simulink model "AD1939_Avalon_Stream_Processing_v1"  (R2018b)
settings: Solver=FixedStepDiscrete  StartTime=0.0  StopTime=stop_time  RelTol=1e-3
InitFcn:
  | DataPlane_callback_init
StopFcn:
  | DataPlane_callback_stop
undefined symbols (not defined in the file or in its folder): F_bits, Ts_system, W_bits
libraries: hdlsllib x18, simulink x5, dspsrcs4 x4, dsphdlfiltering x2
(part 1 of 2)
settings Model: Creator=Ross  LastModifiedBy=trevor
settings OptimizationCC: BlockReduction=off  ConditionallyExecuteInputs=off  DefaultParameterBehavior=Inlined
settings DebuggingCC: AlgebraicLoopMsg=error  SingleTaskRateTransMsg=error  LibraryContextMissingDiagnostic=none
settings HardwareCC: ProdBitPerPointer=32  ProdBitPerSizeT=32  ProdBitPerPtrDiffT=32  ProdLargestAtomicFloat=None  ProdIntDivRoundTo=Undefined  ProdEndianess=Unspecified  ProdWordSize=32  ProdHWDeviceType=ASIC/FPGA->ASIC/FPGA  TargetBitPerLong=64  TargetBitPerPointer=64  TargetBitPerSizeT=64  TargetBitPerPtrDiffT=64  TargetLongLongMode=on  TargetIntDivRoundTo=Zero  TargetEndianess=LittleEndian  TargetWordSize=64  TargetHWDeviceType=Custom Processor->MATLAB Host Computer  ProdEqTarget=off
settings SFSimCC: SimUseLocalCustomCode=off
settings RTWCC: RTWUseLocalCustomCode=off

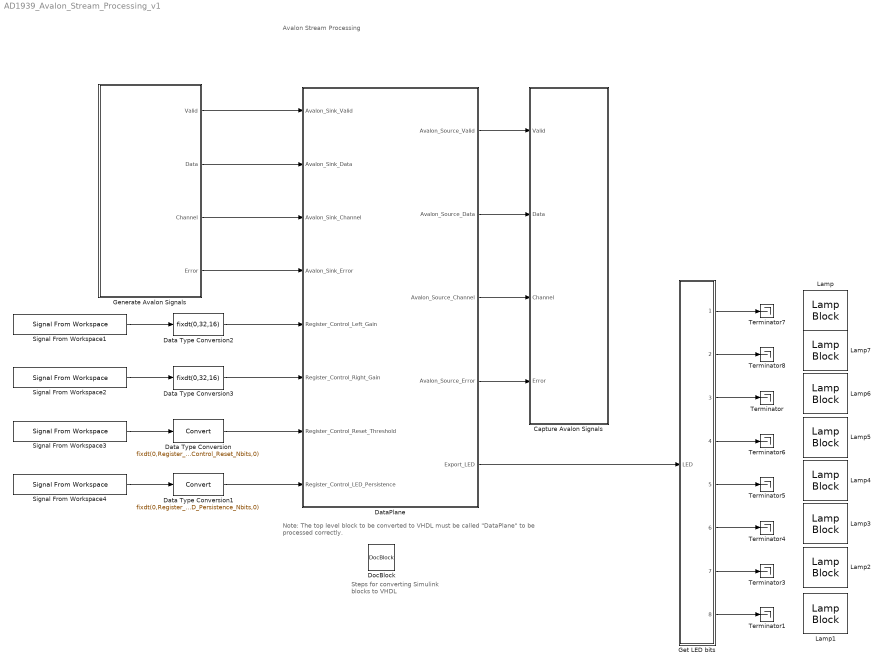
== system AD1939_Avalon_Stream_Processing_v1 ==
  note: Note:  The top level block to be converted to VHDL must be called "DataPlane"
      | to be processed correctly.
  note: Steps for converting
      | Simulink blocks
      | to VHDL
  note: Avalon Stream Processing
  Capture Avalon Signals : Subsystem
  Data Type Conversion : DataTypeConversion  OutDataTypeStr=fixdt(0,Register_Control_Reset_Nbits,0)
  Data Type Conversion1 : DataTypeConversion  OutDataTypeStr=fixdt(0,Register_Control_LED_Persistence_Nbits,0)
  Data Type Conversion2 : DataTypeConversion  OutDataTypeStr=fixdt(0,32,16)
  Data Type Conversion3 : DataTypeConversion  OutDataTypeStr=fixdt(0,32,16)
  DataPlane : Subsystem  TreatAsAtomicUnit=on
  DocBlock : simulink/Model-Wide Utilities/DocBlock  DocumentType=HTML
  Generate Avalon Signals : Subsystem
  Get LED bits : Subsystem
  Lamp : LampBlock  WebBlockId=954
  Lamp1 : LampBlock  WebBlockId=955
  Lamp2 : LampBlock  WebBlockId=956
  Lamp3 : LampBlock  WebBlockId=957
  Lamp4 : LampBlock  WebBlockId=958
  Lamp5 : LampBlock  WebBlockId=959
  Lamp6 : LampBlock  WebBlockId=960
  Lamp7 : LampBlock  WebBlockId=961
  Signal From Workspace1 : dspsrcs4/Signal From Workspace  X=Register_Control_Left_Gain  Ts=Ts_system  nsamps=1  OutputAfterFinalValue=Holding final value  ignoreOrWarnInputAndFrameLengths=off  OutputFrames=off
  Signal From Workspace2 : dspsrcs4/Signal From Workspace  X=Register_Control_Right_Gain  Ts=Ts_system  nsamps=1  OutputAfterFinalValue=Holding final value  ignoreOrWarnInputAndFrameLengths=off  OutputFrames=off
  Signal From Workspace3 : dspsrcs4/Signal From Workspace  X=Register_Control_Reset_Threshold  Ts=Ts_system  nsamps=1  OutputAfterFinalValue=Holding final value  ignoreOrWarnInputAndFrameLengths=off  OutputFrames=off
  Signal From Workspace4 : dspsrcs4/Signal From Workspace  X=Register_Control_LED_Persistence  Ts=Ts_system  nsamps=1  OutputAfterFinalValue=Holding final value  ignoreOrWarnInputAndFrameLengths=off  OutputFrames=off
  Terminator{,1,3..8} (8 alike) : Terminator
  wires:
  Generate Avalon Signals/2(Data) -> DataPlane/2(Avalon_Sink_Data)
  Generate Avalon Signals/1(Valid) -> DataPlane/1(Avalon_Sink_Valid)
  Generate Avalon Signals/3(Channel) -> DataPlane/3(Avalon_Sink_Channel)
  Generate Avalon Signals/4(Error) -> DataPlane/4(Avalon_Sink_Error)
  DataPlane/2(Avalon_Source_Data) -> Capture Avalon Signals/2(Data)
  DataPlane/1(Avalon_Source_Valid) -> Capture Avalon Signals/1(Valid)
  DataPlane/3(Avalon_Source_Channel) -> Capture Avalon Signals/3(Channel)
  DataPlane/4(Avalon_Source_Error) -> Capture Avalon Signals/4(Error)
  Signal From Workspace3/1 -> Data Type Conversion/1
  Signal From Workspace4/1 -> Data Type Conversion1/1
  Data Type Conversion/1 -> DataPlane/7(Register_Control_Reset_Threshold)
  Data Type Conversion1/1 -> DataPlane/8(Register_Control_LED_Persistence)
  Get LED bits/7(LED_1) -> Terminator3/1
  Get LED bits/4(LED_4) -> Terminator6/1
  Get LED bits/1(LED_7) -> Terminator7/1
  Get LED bits/6(LED_2) -> Terminator4/1
  Get LED bits/2(LED_6) -> Terminator8/1
  Get LED bits/8(LED_0) -> Terminator1/1
  Get LED bits/5(LED_3) -> Terminator5/1
  Get LED bits/3(LED_5) -> Terminator/1
  DataPlane/5(Export_LED) -> Get LED bits/1(LED)
  Signal From Workspace1/1 -> Data Type Conversion2/1
  Signal From Workspace2/1 -> Data Type Conversion3/1
  Data Type Conversion2/1 -> DataPlane/5(Register_Control_Left_Gain)
  Data Type Conversion3/1 -> DataPlane/6(Register_Control_Right_Gain)

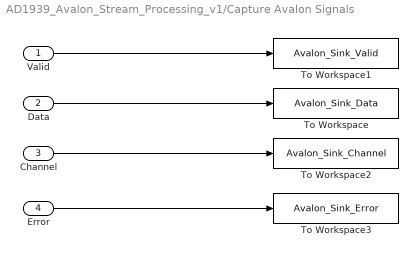
== system AD1939_Avalon_Stream_Processing_v1/Capture Avalon Signals ==
  Valid : Inport
  Data : Inport  Port=2
  Channel : Inport  Port=3
  Error : Inport  Port=4
  To Workspace : ToWorkspace  VariableName=Avalon_Sink_Data  SaveFormat=Timeseries  SampleTime=-1
  To Workspace1 : ToWorkspace  VariableName=Avalon_Sink_Valid  SaveFormat=Timeseries  SampleTime=-1
  To Workspace2 : ToWorkspace  VariableName=Avalon_Sink_Channel  SaveFormat=Timeseries  SampleTime=-1
  To Workspace3 : ToWorkspace  VariableName=Avalon_Sink_Error  SaveFormat=Timeseries  SampleTime=-1
  wires:
  Data/1 -> To Workspace/1
  Valid/1 -> To Workspace1/1
  Error/1 -> To Workspace3/1
  Channel/1 -> To Workspace2/1

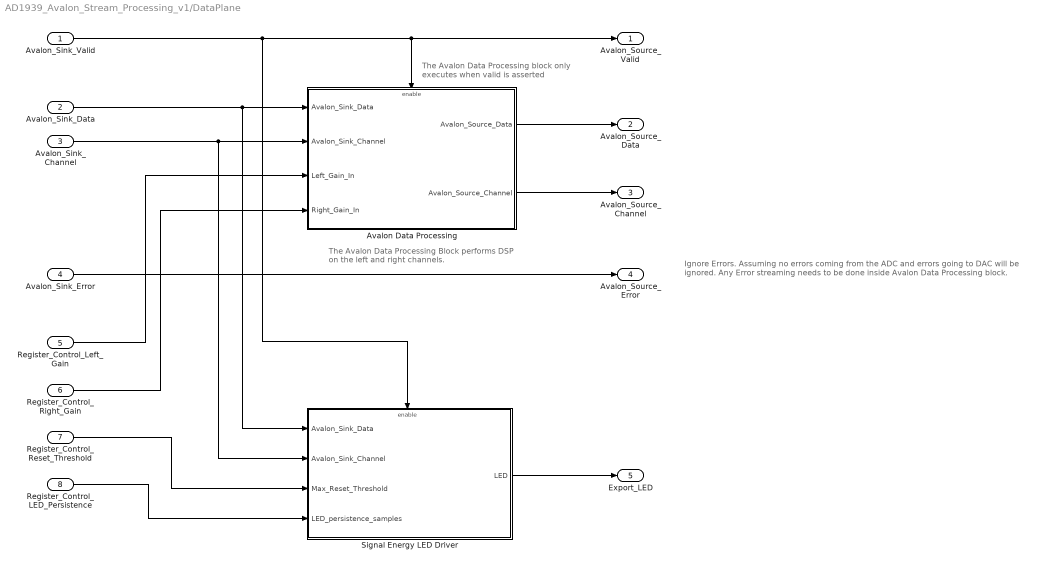
== system AD1939_Avalon_Stream_Processing_v1/DataPlane ==
  note: The Avalon Data Processing Block
      | performs DSP on the left and right channels.
  note: The Avalon Data Processing block
      | only executes when valid is asserted
  note: Ignore Errors.
      | Assuming no errors coming from the ADC and errors going to DAC will be ignored.
      | Any Error streaming needs to be done inside Avalon Data Processing block.
  Avalon_Sink_Valid : Inport
  Avalon_Sink_Data : Inport  Port=2
  Avalon_Sink_Channel : Inport  Port=3
  Avalon_Sink_Error : Inport  Port=4
  Register_Control_Left_Gain : Inport  Port=5
  Register_Control_Right_Gain : Inport  Port=6
  Register_Control_Reset_Threshold : Inport  Port=7
  Register_Control_LED_Persistence : Inport  Port=8
  Avalon Data Processing : Subsystem  TreatAsAtomicUnit=on
  Signal Energy LED Driver : Subsystem  TreatAsAtomicUnit=on
  Avalon_Source_Valid : Outport
  Avalon_Source_Data : Outport  Port=2
  Avalon_Source_Channel : Outport  Port=3
  Avalon_Source_Error : Outport  Port=4
  Export_LED : Outport  Port=5  InitialOutput=0
  wires:
  Avalon_Sink_Channel/1 -> Signal Energy LED Driver/2(Avalon_Sink_Channel), Avalon Data Processing/2(Avalon_Sink_Channel)
  Avalon_Sink_Error/1 -> Avalon_Source_Error/1
  Avalon Data Processing/1(Avalon_Source_Data) -> Avalon_Source_Data/1
  Avalon_Sink_Valid/1 -> Signal Energy LED Driver/Enable, Avalon Data Processing/Enable, Avalon_Source_Valid/1
  Avalon_Sink_Data/1 -> Signal Energy LED Driver/1(Avalon_Sink_Data), Avalon Data Processing/1(Avalon_Sink_Data)
  Avalon Data Processing/2(Avalon_Source_Channel) -> Avalon_Source_Channel/1
  Register_Control_Right_Gain/1 -> Avalon Data Processing/4(Right_Gain_In)
  Register_Control_Left_Gain/1 -> Avalon Data Processing/3(Left_Gain_In)
  Signal Energy LED Driver/1(LED) -> Export_LED/1
  Register_Control_Reset_Threshold/1 -> Signal Energy LED Driver/3(Max_Reset_Threshold)
  Register_Control_LED_Persistence/1 -> Signal Energy LED Driver/4(LED_persistence_samples)

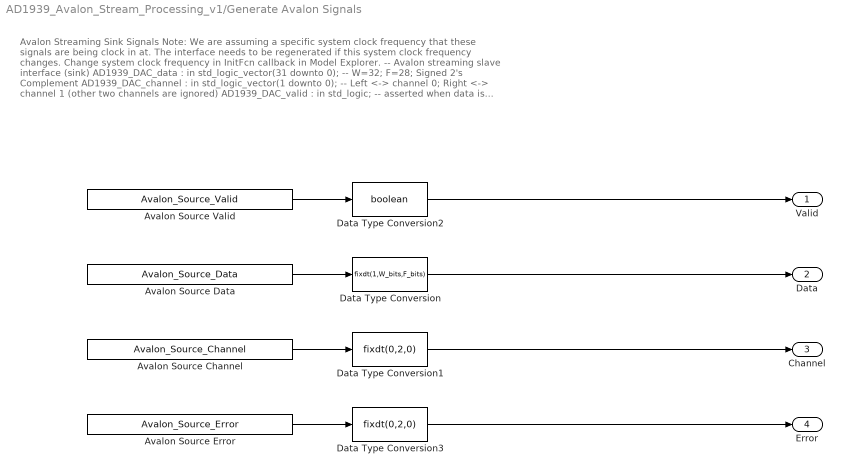
== system AD1939_Avalon_Stream_Processing_v1/Generate Avalon Signals ==
  note: Avalon Streaming Sink Signals
      | Note: We are assuming a specific system clock frequency that these signals are being clock in at.
      | The interface needs to be regenerated if this system clock frequency changes. Change system clock frequency in InitFcn callback in Model Explorer.
      |
      | -- Avalon streaming slave interface (sink)
      | AD1939_DAC_data : in std_logic_vector(31 downto 0); -- W=32; F=28; Signed 2's Complement
      | AD1939_DAC_channel : in std_logic_vector(1 downto 0); -- Left <-> channel 0; Right <-> channel 1 (other two channels are ignored)
      | AD1939_DAC_valid : in std_logic; -- asserted when data is valid
      | AD1939_DAC_error : in std_logic_vector(1 downto 0) -- error channel is ignored, assumed to be error free at this point
  Avalon Source Channel : FromWorkspace  VariableName=Avalon_Source_Channel  OutDataTypeStr=double  SampleTime=Ts_system
  "Avalon Source Data " : FromWorkspace  VariableName=Avalon_Source_Data  OutDataTypeStr=double  SampleTime=Ts_system
  Avalon Source Error : FromWorkspace  VariableName=Avalon_Source_Error  OutDataTypeStr=double  SampleTime=Ts_system
  Avalon Source Valid : FromWorkspace  VariableName=Avalon_Source_Valid  OutDataTypeStr=double  SampleTime=Ts_system
  Data Type Conversion : DataTypeConversion  OutDataTypeStr=fixdt(1,W_bits,F_bits)
  Data Type Conversion1 : DataTypeConversion  OutDataTypeStr=fixdt(0,2,0)
  Data Type Conversion2 : DataTypeConversion  OutDataTypeStr=boolean
  Data Type Conversion3 : DataTypeConversion  OutDataTypeStr=fixdt(0,2,0)
  Valid : Outport
  Data : Outport  Port=2
  Channel : Outport  Port=3
  Error : Outport  Port=4
  wires:
  Data Type Conversion1/1 -> Channel/1
  Data Type Conversion2/1 -> Valid/1
  Avalon Source Error/1 -> Data Type Conversion3/1
  Data Type Conversion/1 -> Data/1
  Avalon Source Valid/1 -> Data Type Conversion2/1
  Data Type Conversion3/1 -> Error/1
  Avalon Source Channel/1 -> Data Type Conversion1/1
  "Avalon Source Data "/1 -> Data Type Conversion/1

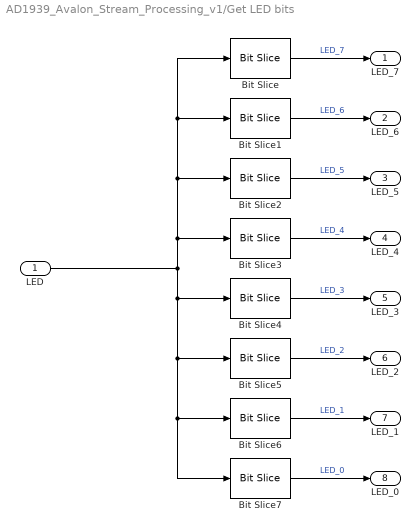
== system AD1939_Avalon_Stream_Processing_v1/Get LED bits ==
  LED : Inport
  Bit Slice : hdlsllib/Logic and Bit Operations/Bit Slice  lidx=7  ridx=7
  Bit Slice1 : hdlsllib/Logic and Bit Operations/Bit Slice  lidx=6  ridx=6
  Bit Slice2 : hdlsllib/Logic and Bit Operations/Bit Slice  lidx=5  ridx=5
  Bit Slice3 : hdlsllib/Logic and Bit Operations/Bit Slice  lidx=4  ridx=4
  Bit Slice4 : hdlsllib/Logic and Bit Operations/Bit Slice  lidx=3  ridx=3
  Bit Slice5 : hdlsllib/Logic and Bit Operations/Bit Slice  lidx=2  ridx=2
  Bit Slice6 : hdlsllib/Logic and Bit Operations/Bit Slice  lidx=1  ridx=1
  Bit Slice7 : hdlsllib/Logic and Bit Operations/Bit Slice  lidx=0  ridx=0
  LED_7 : Outport
  LED_6 : Outport  Port=2
  LED_5 : Outport  Port=3
  LED_4 : Outport  Port=4
  LED_3 : Outport  Port=5
  LED_2 : Outport  Port=6
  LED_1 : Outport  Port=7
  LED_0 : Outport  Port=8
  wires:
  Bit Slice6/1 -> LED_1/1  "LED_1"
  LED/1 -> Bit Slice4/1, Bit Slice5/1, Bit Slice6/1, Bit Slice7/1, Bit Slice3/1, Bit Slice/1, Bit Slice1/1, Bit Slice2/1
  Bit Slice1/1 -> LED_6/1  "LED_6"
  Bit Slice/1 -> LED_7/1  "LED_7"
  Bit Slice7/1 -> LED_0/1  "LED_0"
  Bit Slice5/1 -> LED_2/1  "LED_2"
  Bit Slice2/1 -> LED_5/1  "LED_5"
  Bit Slice3/1 -> LED_4/1  "LED_4"
  Bit Slice4/1 -> LED_3/1  "LED_3"

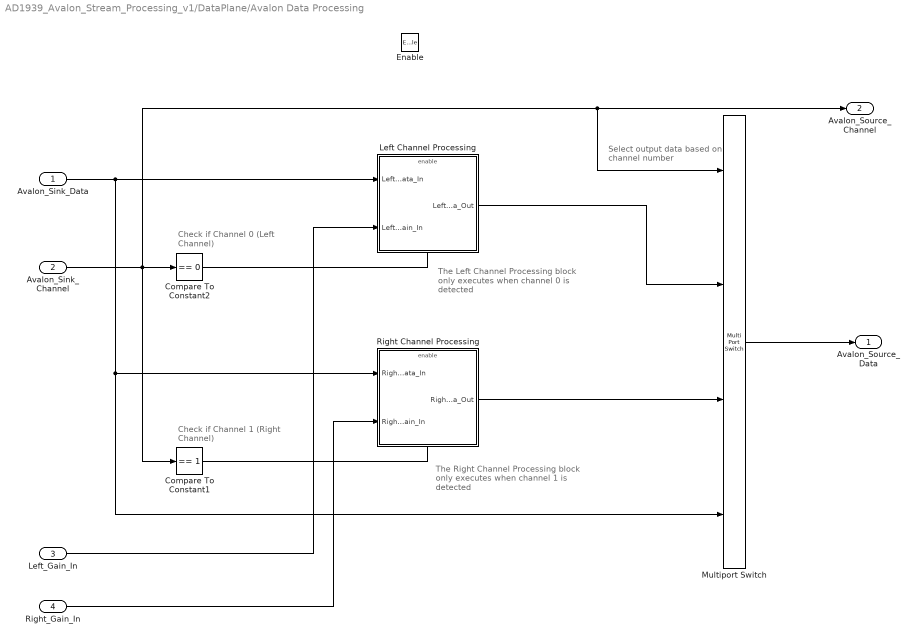
== system AD1939_Avalon_Stream_Processing_v1/DataPlane/Avalon Data Processing ==
  note: Select output data
      | based on channel number
  note: Check if Channel 0
      | (Left Channel)
  note: The Left Channel Processing block
      | only executes when channel 0
      | is detected
  note: The Right Channel Processing block
      | only executes when channel 1
      | is detected
  note: Check if Channel 1
      | (Right Channel)
  Avalon_Sink_Data : Inport
  Avalon_Sink_Channel : Inport  Port=2
  Left_Gain_In : Inport  Port=3
  Right_Gain_In : Inport  Port=4
  Enable : EnablePort
  Compare To Constant1 : simulink/Logic and Bit Operations/Compare To Constant  relop===  const=1  OutDataTypeStr=boolean
  Compare To Constant2 : simulink/Logic and Bit Operations/Compare To Constant  relop===  const=0  OutDataTypeStr=boolean
  Left Channel Processing : Subsystem  TreatAsAtomicUnit=on
  Multiport Switch : MultiPortSwitch  DataPortOrder=Zero-based contiguous  zeroidx=on
  Right Channel Processing : Subsystem  TreatAsAtomicUnit=on
  Avalon_Source_Data : Outport  InitialOutput=0
  Avalon_Source_Channel : Outport  Port=2  InitialOutput=0
  wires:
  Avalon_Sink_Channel/1 -> Avalon_Source_Channel/1, Multiport Switch/1, Compare To Constant1/1, Compare To Constant2/1
  Compare To Constant2/1 -> Left Channel Processing/Enable
  Compare To Constant1/1 -> Right Channel Processing/Enable
  Avalon_Sink_Data/1 -> Multiport Switch/4, Right Channel Processing/1(Right_Data_In), Left Channel Processing/1(Left_Data_In)
  Left Channel Processing/1("Left_Data_Out ") -> Multiport Switch/2
  Right Channel Processing/1("Right_Data_Out ") -> Multiport Switch/3
  Multiport Switch/1 -> Avalon_Source_Data/1
  Left_Gain_In/1 -> Left Channel Processing/2(Left_Gain_In)
  Right_Gain_In/1 -> Right Channel Processing/2(Right_Gain_In)

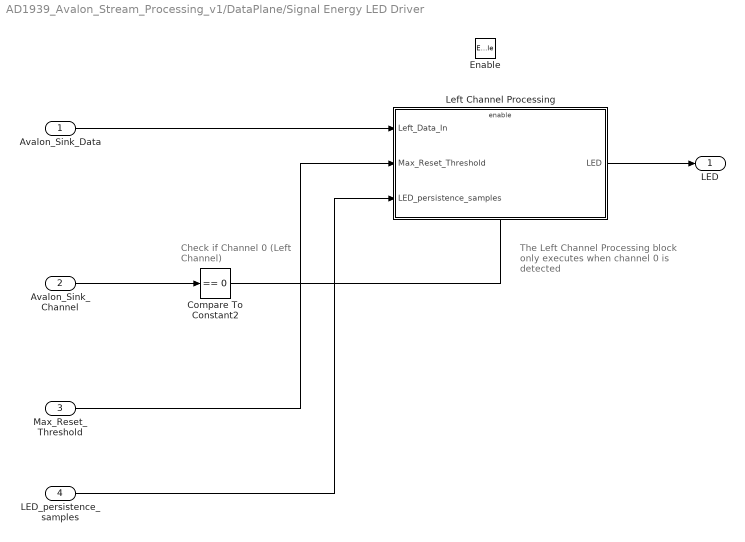
== system AD1939_Avalon_Stream_Processing_v1/DataPlane/Signal Energy LED Driver ==
  note: The Left Channel Processing block
      | only executes when channel 0
      | is detected
  note: Check if Channel 0
      | (Left Channel)
  Avalon_Sink_Data : Inport
  Avalon_Sink_Channel : Inport  Port=2
  Max_Reset_Threshold : Inport  Port=3
  LED_persistence_samples : Inport  Port=4
  Enable : EnablePort
  Compare To Constant2 : simulink/Logic and Bit Operations/Compare To Constant  relop===  const=0  OutDataTypeStr=boolean
  Left Channel Processing : Subsystem  TreatAsAtomicUnit=on
  LED : Outport  InitialOutput=0
  wires:
  Max_Reset_Threshold/1 -> Left Channel Processing/2(Max_Reset_Threshold)
  LED_persistence_samples/1 -> Left Channel Processing/3(LED_persistence_samples)
  Avalon_Sink_Channel/1 -> Compare To Constant2/1
  Left Channel Processing/1(LED) -> LED/1
  Avalon_Sink_Data/1 -> Left Channel Processing/1(Left_Data_In)
  Compare To Constant2/1 -> Left Channel Processing/Enable

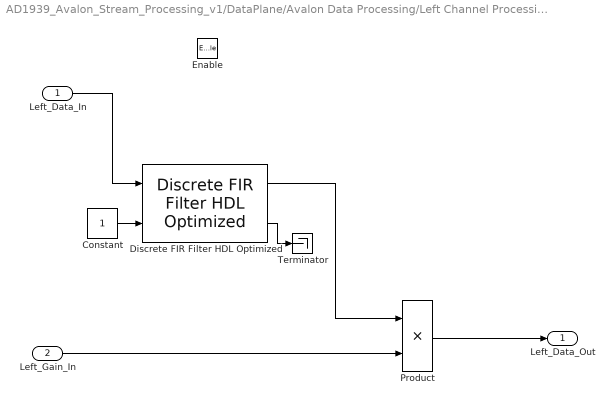
== system AD1939_Avalon_Stream_Processing_v1/DataPlane/Avalon Data Processing/Left Channel Processing ==
  Left_Data_In : Inport
  Left_Gain_In : Inport  Port=2
  Enable : EnablePort
  Constant : Constant  OutDataTypeStr=boolean  SampleTime=Ts_system
  Discrete FIR Filter HDL Optimized : dsphdlfiltering/Discrete FIR Filter HDL Optimized  Numerator=fir1(30,2/24,'low')  FilterStructure=Direct form transposed  Sharing=off  SharingFactor=2  SimulateUsing=Code generation  roundingMode=Floor  overflowMode=off  CoefficientsDataTypeStr=Inherit: Same word length as input  CoefficientsMin=[]  CoefficientsMax=[]  OutputDataTypeStr=fixdt(1,W_bits,F_bits)  OutputMin=[]  OutputMax=[]  ResetInputPort=off  HDLGlobalReset=off
      settings: SourceProductName=DSP System Toolbox  SourceProductBaseCode=DS
  Product : Product  OutDataTypeStr=Inherit: Same as first input
  Terminator : Terminator
  "Left_Data_Out " : Outport  InitialOutput=0
  wires:
  Left_Data_In/1 -> Discrete FIR Filter HDL Optimized/1
  Discrete FIR Filter HDL Optimized/1 -> Product/1
  Product/1 -> "Left_Data_Out "/1
  Left_Gain_In/1 -> Product/2
  Discrete FIR Filter HDL Optimized/2 -> Terminator/1
  Constant/1 -> Discrete FIR Filter HDL Optimized/2

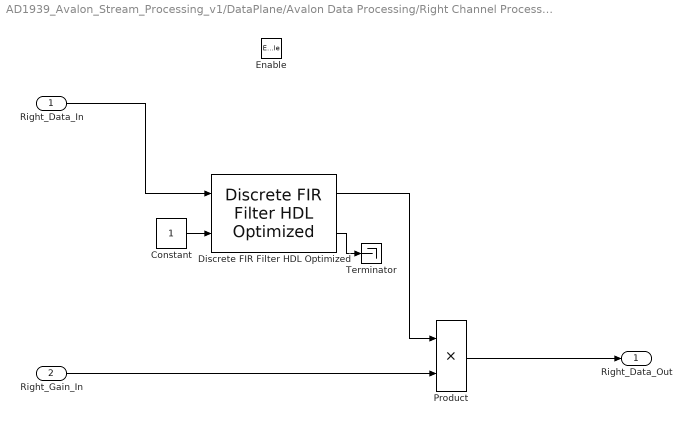
== system AD1939_Avalon_Stream_Processing_v1/DataPlane/Avalon Data Processing/Right Channel Processing ==
  Right_Data_In : Inport
  Right_Gain_In : Inport  Port=2
  Enable : EnablePort
  Constant : Constant  OutDataTypeStr=boolean  SampleTime=Ts_system
  Discrete FIR Filter HDL Optimized : dsphdlfiltering/Discrete FIR Filter HDL Optimized  Numerator=fir1(30,2/24,'high')  FilterStructure=Direct form transposed  Sharing=off  SharingFactor=2  SimulateUsing=Code generation  roundingMode=Floor  overflowMode=off  CoefficientsDataTypeStr=Inherit: Same word length as input  CoefficientsMin=[]  CoefficientsMax=[]  OutputDataTypeStr=fixdt(1,W_bits,F_bits)  OutputMin=[]  OutputMax=[]  ResetInputPort=off  HDLGlobalReset=off
      settings: SourceProductName=DSP System Toolbox  SourceProductBaseCode=DS
  Product : Product  OutDataTypeStr=Inherit: Same as first input
  Terminator : Terminator
  "Right_Data_Out " : Outport  InitialOutput=0
  wires:
  Right_Gain_In/1 -> Product/2
  Product/1 -> "Right_Data_Out "/1
  Discrete FIR Filter HDL Optimized/1 -> Product/1
  Right_Data_In/1 -> Discrete FIR Filter HDL Optimized/1
  Constant/1 -> Discrete FIR Filter HDL Optimized/2
  Discrete FIR Filter HDL Optimized/2 -> Terminator/1

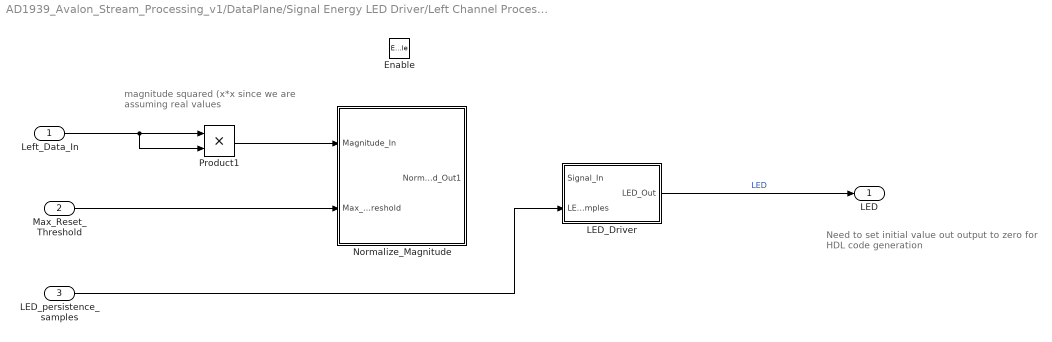
== system AD1939_Avalon_Stream_Processing_v1/DataPlane/Signal Energy LED Driver/Left Channel Processing ==
  note: magnitude squared
      | (x*x since we are assuming real values
  note: Need to set initial value out output to zero
      | for HDL code generation
  Left_Data_In : Inport
  Max_Reset_Threshold : Inport  Port=2
  LED_persistence_samples : Inport  Port=3
  Enable : EnablePort
  LED_Driver : Subsystem
  Normalize_Magnitude : Subsystem
  Product1 : Product  OutDataTypeStr=fixdt(1,W_bits,F_bits)
  LED : Outport  InitialOutput=0
  wires:
  Left_Data_In/1 -> Product1/2, Product1/1
  LED_persistence_samples/1 -> LED_Driver/2(LED_persistence_samples)
  ? -> LED_Driver/1(Signal_In)
  Max_Reset_Threshold/1 -> Normalize_Magnitude/2(Max_Reset_Threshold)
  Product1/1 -> Normalize_Magnitude/1(Magnitude_In)
  LED_Driver/1(LED_Out) -> LED/1  "LED"

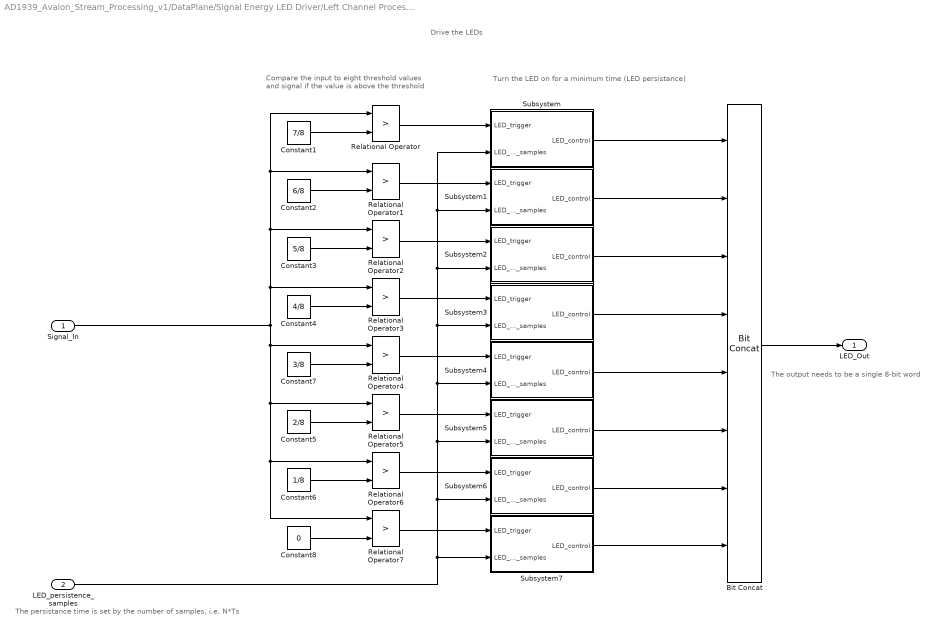
== system AD1939_Avalon_Stream_Processing_v1/DataPlane/Signal Energy LED Driver/Left Channel Processing/LED_Driver ==
  note: The output needs to be a single 8-bit word
  note: The persistance time is set by the number of samples, i.e. N*Ts
  note: Turn the LED on for a minimum time (LED persistance)
  note: Compare the input to eight threshold values
      | and signal if the value is above the threshold
  note: Drive the LEDs
  Signal_In : Inport
  LED_persistence_samples : Inport  Port=2
  Bit Concat : hdlsllib/Logic and Bit Operations/Bit Concat  numInputs=8
      settings: SourceProductName=HDL Coder  SourceProductBaseCode=HD
  Constant1 : Constant  Value=7/8  OutDataTypeStr=fixdt(1,32,28)  SampleTime=Ts_system
  Constant2 : Constant  Value=6/8  OutDataTypeStr=fixdt(1,32,28)  SampleTime=Ts_system
  Constant3 : Constant  Value=5/8  OutDataTypeStr=fixdt(1,32,28)  SampleTime=Ts_system
  Constant4 : Constant  Value=4/8  OutDataTypeStr=fixdt(1,32,28)  SampleTime=Ts_system
  Constant5 : Constant  Value=2/8  OutDataTypeStr=fixdt(1,32,28)  SampleTime=Ts_system
  Constant6 : Constant  Value=1/8  OutDataTypeStr=fixdt(1,32,28)  SampleTime=Ts_system
  Constant7 : Constant  Value=3/8  OutDataTypeStr=fixdt(1,32,28)  SampleTime=Ts_system
  Constant8 : Constant  Value=0  OutDataTypeStr=fixdt(1,32,28)  SampleTime=Ts_system
  Relational Operator{,1..7} (8 alike) : RelationalOperator  Operator=>  OutDataTypeStr=boolean  RndMeth=Nearest
  Subsystem : Subsystem
  Subsystem1 : Subsystem
  Subsystem2 : Subsystem
  Subsystem3 : Subsystem
  Subsystem4 : Subsystem
  Subsystem5 : Subsystem
  Subsystem6 : Subsystem
  Subsystem7 : Subsystem
  LED_Out : Outport
  wires:
  Constant3/1 -> Relational Operator2/2
  Constant6/1 -> Relational Operator6/2
  Constant5/1 -> Relational Operator5/2
  Constant7/1 -> Relational Operator4/2
  Constant8/1 -> Relational Operator7/2
  Signal_In/1 -> Relational Operator/1, Relational Operator1/1, Relational Operator2/1, Relational Operator3/1, Relational Operator4/1, Relational Operator5/1, Relational Operator6/1, Relational Operator7/1
  Constant2/1 -> Relational Operator1/2
  Constant1/1 -> Relational Operator/2
  Constant4/1 -> Relational Operator3/2
  Bit Concat/1 -> LED_Out/1
  Relational Operator/1 -> Subsystem/1(LED_trigger)
  LED_persistence_samples/1 -> Subsystem7/2(LED_persistence_samples), Subsystem6/2(LED_persistence_samples), Subsystem5/2(LED_persistence_samples), Subsystem4/2(LED_persistence_samples), Subsystem3/2(LED_persistence_samples), Subsystem2/2(LED_persistence_samples), Subsystem1/2(LED_persistence_samples), Subsystem/2(LED_persistence_samples)
  Subsystem/1("LED_control ") -> Bit Concat/1
  Subsystem1/1("LED_control ") -> Bit Concat/2
  Subsystem2/1("LED_control ") -> Bit Concat/3
  Subsystem3/1("LED_control ") -> Bit Concat/4
  Subsystem4/1("LED_control ") -> Bit Concat/5
  Subsystem5/1("LED_control ") -> Bit Concat/6
  Subsystem6/1("LED_control ") -> Bit Concat/7
  Subsystem7/1("LED_control ") -> Bit Concat/8
  Relational Operator1/1 -> Subsystem1/1(LED_trigger)
  Relational Operator2/1 -> Subsystem2/1(LED_trigger)
  Relational Operator3/1 -> Subsystem3/1(LED_trigger)
  Relational Operator4/1 -> Subsystem4/1(LED_trigger)
  Relational Operator5/1 -> Subsystem5/1(LED_trigger)
  Relational Operator6/1 -> Subsystem6/1(LED_trigger)
  Relational Operator7/1 -> Subsystem7/1(LED_trigger)

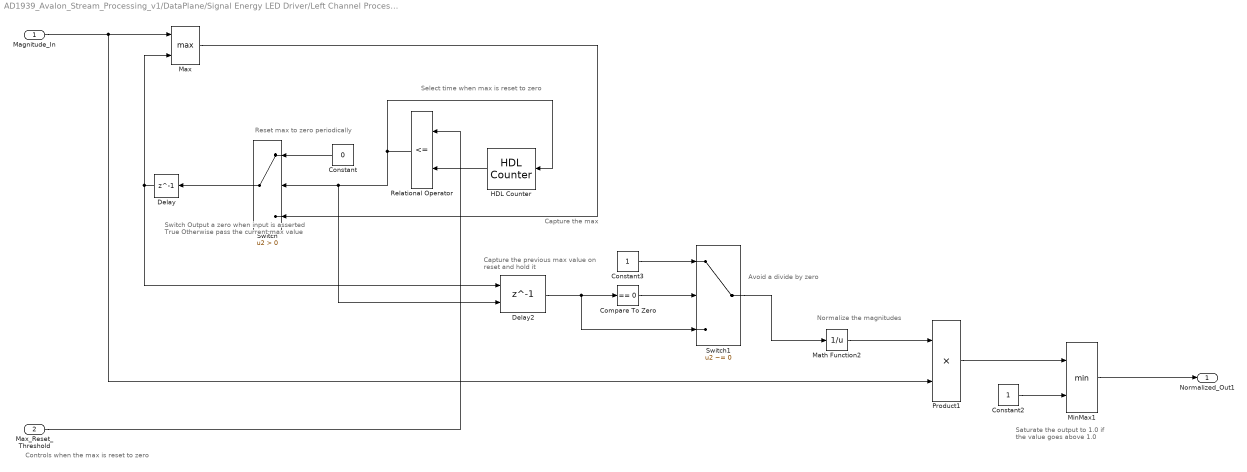
== system AD1939_Avalon_Stream_Processing_v1/DataPlane/Signal Energy LED Driver/Left Channel Processing/Normalize_Magnitude ==
  note: Controls when the max is reset to zero
  note: Select time when max is reset to zero
  note: Switch
      | Output a zero when input is asserted True
      | Otherwise pass the current max value
  note: Capture the max
  note: Reset max to zero periodically
  note: Normalize the magnitudes
  note: Capture the previous max value
      | on reset and hold it
  note: Avoid a divide by zero
  note: Saturate the output to 1.0
      | if the value goes above 1.0
  Magnitude_In : Inport
  Max_Reset_Threshold : Inport  Port=2
  Compare To Zero : simulink/Logic and Bit Operations/Compare To Zero  relop===  OutDataTypeStr=boolean
  Constant : Constant  Value=0  OutDataTypeStr=fixdt(1,32,28)  SampleTime=Ts_system
  Constant2 : Constant  OutDataTypeStr=fixdt(1,W_bits,F_bits)  SampleTime=Ts_system
  Constant3 : Constant  OutDataTypeStr=fixdt(1,W_bits,F_bits)  SampleTime=Ts_system
  Delay : Delay  DelayLength=1
  Delay2 : Delay  DelayLength=1  ShowEnablePort=on
      settings: InputPortMap=u0,e6
  "HDL Counter " : hdlsllib/Sources/HDL Counter  CountType=Free running  CountInit=0  CountStep=1  CountMax=25  CountFromType=Initial value  CountFrom=0  CountResetPort=on  CountLoadPort=off  CountEnbPort=off  CountDirPort=off  CountDataType=Unsigned  CountWordLen=Register_Control_Reset_Nbits  CountFracLen=0  CountSampTime=1
      settings: SourceProductBaseCode=HD
  Math Function2 : Math  Operator=reciprocal  RndMeth=Zero  SaturateOnIntegerOverflow=on
  Max : MinMax  Function=max  Inputs=2
  MinMax1 : MinMax  Inputs=2
  Product1 : Product  OutDataTypeStr=Inherit: Same as first input
  Relational Operator : RelationalOperator  Operator=<=  OutDataTypeStr=boolean  RndMeth=Nearest
  Switch : Switch  Criteria=u2 > Threshold
  Switch1 : Switch  Criteria=u2 ~= 0
  Normalized_Out1 : Outport
  wires:
  Max/1 -> Switch/3
  Delay/1 -> Delay2/1, Max/2
  Switch/1 -> Delay/1
  Relational Operator/1 -> "HDL Counter "/1, Delay2/2, Switch/2
  Magnitude_In/1 -> Product1/2, Max/1
  Constant/1 -> Switch/1
  "HDL Counter "/1 -> Relational Operator/2
  Max_Reset_Threshold/1 -> Relational Operator/1
  Constant3/1 -> Switch1/1
  Compare To Zero/1 -> Switch1/2
  Switch1/1 -> Math Function2/1
  Delay2/1 -> Switch1/3, Compare To Zero/1
  Math Function2/1 -> Product1/1
  MinMax1/1 -> Normalized_Out1/1
  Product1/1 -> MinMax1/1
  Constant2/1 -> MinMax1/2

== system AD1939_Avalon_Stream_Processing_v1/DataPlane/Signal Energy LED Driver/Left Channel Processing/LED_Driver/Subsystem ==
  note: Don't start counter
      | as long as LED_trigger is asserted
  LED_trigger : Inport
  LED_persistence_samples : Inport  Port=2
  Chart : Stateflow chart  TreatAsAtomicUnit=on
  "HDL Counter " : hdlsllib/Sources/HDL Counter  CountType=Free running  CountInit=0  CountStep=1  CountMax=25  CountFromType=Initial value  CountFrom=0  CountResetPort=on  CountLoadPort=off  CountEnbPort=off  CountDirPort=off  CountDataType=Unsigned  CountWordLen=Register_Control_LED_Persistence_Nbits  CountFracLen=0  CountSampTime=1
      settings: SourceProductBaseCode=HD
  Logical Operator : Logic  Operator=OR  AllPortsSameDT=off  OutDataTypeStr=boolean
  Relational Operator8 : RelationalOperator  Operator=<=  OutDataTypeStr=boolean  RndMeth=Nearest
  "LED_control " : Outport
  wires:
  Relational Operator8/1 -> Chart/2(count_reached)
  LED_trigger/1 -> Logical Operator/2, Chart/1(LED_trigger)
  Chart/1(LED_signal) -> "LED_control "/1
  "HDL Counter "/1 -> Relational Operator8/2
  LED_persistence_samples/1 -> Relational Operator8/1
  Chart/2(counter_reset) -> Logical Operator/1
  Logical Operator/1 -> "HDL Counter "/1

== system AD1939_Avalon_Stream_Processing_v1/DataPlane/Signal Energy LED Driver/Left Channel Processing/LED_Driver/Subsystem1 ==
  note: Don't start counter
      | as long as LED_trigger is asserted
  LED_trigger : Inport
  LED_persistence_samples : Inport  Port=2
  Chart : Stateflow chart  TreatAsAtomicUnit=on
  "HDL Counter " : hdlsllib/Sources/HDL Counter  CountType=Free running  CountInit=0  CountStep=1  CountMax=25  CountFromType=Initial value  CountFrom=0  CountResetPort=on  CountLoadPort=off  CountEnbPort=off  CountDirPort=off  CountDataType=Unsigned  CountWordLen=Register_Control_LED_Persistence_Nbits  CountFracLen=0  CountSampTime=1
      settings: SourceProductBaseCode=HD
  Logical Operator : Logic  Operator=OR  AllPortsSameDT=off  OutDataTypeStr=boolean
  Relational Operator8 : RelationalOperator  Operator=<=  OutDataTypeStr=boolean  RndMeth=Nearest
  "LED_control " : Outport
  wires:
  Relational Operator8/1 -> Chart/2(count_reached)
  LED_trigger/1 -> Logical Operator/2, Chart/1(LED_trigger)
  Chart/1(LED_signal) -> "LED_control "/1
  "HDL Counter "/1 -> Relational Operator8/2
  LED_persistence_samples/1 -> Relational Operator8/1
  Chart/2(counter_reset) -> Logical Operator/1
  Logical Operator/1 -> "HDL Counter "/1

== system AD1939_Avalon_Stream_Processing_v1/DataPlane/Signal Energy LED Driver/Left Channel Processing/LED_Driver/Subsystem2 ==
  note: Don't start counter
      | as long as LED_trigger is asserted
  LED_trigger : Inport
  LED_persistence_samples : Inport  Port=2
  Chart : Stateflow chart  TreatAsAtomicUnit=on
  "HDL Counter " : hdlsllib/Sources/HDL Counter  CountType=Free running  CountInit=0  CountStep=1  CountMax=25  CountFromType=Initial value  CountFrom=0  CountResetPort=on  CountLoadPort=off  CountEnbPort=off  CountDirPort=off  CountDataType=Unsigned  CountWordLen=Register_Control_LED_Persistence_Nbits  CountFracLen=0  CountSampTime=1
      settings: SourceProductBaseCode=HD
  Logical Operator : Logic  Operator=OR  AllPortsSameDT=off  OutDataTypeStr=boolean
  Relational Operator8 : RelationalOperator  Operator=<=  OutDataTypeStr=boolean  RndMeth=Nearest
  "LED_control " : Outport
  wires:
  Relational Operator8/1 -> Chart/2(count_reached)
  LED_trigger/1 -> Logical Operator/2, Chart/1(LED_trigger)
  Chart/1(LED_signal) -> "LED_control "/1
  "HDL Counter "/1 -> Relational Operator8/2
  LED_persistence_samples/1 -> Relational Operator8/1
  Chart/2(counter_reset) -> Logical Operator/1
  Logical Operator/1 -> "HDL Counter "/1

== system AD1939_Avalon_Stream_Processing_v1/DataPlane/Signal Energy LED Driver/Left Channel Processing/LED_Driver/Subsystem3 ==
  note: Don't start counter
      | as long as LED_trigger is asserted
  LED_trigger : Inport
  LED_persistence_samples : Inport  Port=2
  Chart : Stateflow chart  TreatAsAtomicUnit=on
  "HDL Counter " : hdlsllib/Sources/HDL Counter  CountType=Free running  CountInit=0  CountStep=1  CountMax=25  CountFromType=Initial value  CountFrom=0  CountResetPort=on  CountLoadPort=off  CountEnbPort=off  CountDirPort=off  CountDataType=Unsigned  CountWordLen=Register_Control_LED_Persistence_Nbits  CountFracLen=0  CountSampTime=1
      settings: SourceProductBaseCode=HD
  Logical Operator : Logic  Operator=OR  AllPortsSameDT=off  OutDataTypeStr=boolean
  Relational Operator8 : RelationalOperator  Operator=<=  OutDataTypeStr=boolean  RndMeth=Nearest
  "LED_control " : Outport
  wires:
  Relational Operator8/1 -> Chart/2(count_reached)
  LED_trigger/1 -> Logical Operator/2, Chart/1(LED_trigger)
  Chart/1(LED_signal) -> "LED_control "/1
  "HDL Counter "/1 -> Relational Operator8/2
  LED_persistence_samples/1 -> Relational Operator8/1
  Chart/2(counter_reset) -> Logical Operator/1
  Logical Operator/1 -> "HDL Counter "/1

== system AD1939_Avalon_Stream_Processing_v1/DataPlane/Signal Energy LED Driver/Left Channel Processing/LED_Driver/Subsystem4 ==
  note: Don't start counter
      | as long as LED_trigger is asserted
  LED_trigger : Inport
  LED_persistence_samples : Inport  Port=2
  Chart : Stateflow chart  TreatAsAtomicUnit=on
  "HDL Counter " : hdlsllib/Sources/HDL Counter  CountType=Free running  CountInit=0  CountStep=1  CountMax=25  CountFromType=Initial value  CountFrom=0  CountResetPort=on  CountLoadPort=off  CountEnbPort=off  CountDirPort=off  CountDataType=Unsigned  CountWordLen=Register_Control_LED_Persistence_Nbits  CountFracLen=0  CountSampTime=1
      settings: SourceProductBaseCode=HD
  Logical Operator : Logic  Operator=OR  AllPortsSameDT=off  OutDataTypeStr=boolean
  Relational Operator8 : RelationalOperator  Operator=<=  OutDataTypeStr=boolean  RndMeth=Nearest
  "LED_control " : Outport
  wires:
  Relational Operator8/1 -> Chart/2(count_reached)
  LED_trigger/1 -> Logical Operator/2, Chart/1(LED_trigger)
  Chart/1(LED_signal) -> "LED_control "/1
  "HDL Counter "/1 -> Relational Operator8/2
  LED_persistence_samples/1 -> Relational Operator8/1
  Chart/2(counter_reset) -> Logical Operator/1
  Logical Operator/1 -> "HDL Counter "/1

== system AD1939_Avalon_Stream_Processing_v1/DataPlane/Signal Energy LED Driver/Left Channel Processing/LED_Driver/Subsystem5 ==
  note: Don't start counter
      | as long as LED_trigger is asserted
  LED_trigger : Inport
  LED_persistence_samples : Inport  Port=2
  Chart : Stateflow chart  TreatAsAtomicUnit=on
  "HDL Counter " : hdlsllib/Sources/HDL Counter  CountType=Free running  CountInit=0  CountStep=1  CountMax=25  CountFromType=Initial value  CountFrom=0  CountResetPort=on  CountLoadPort=off  CountEnbPort=off  CountDirPort=off  CountDataType=Unsigned  CountWordLen=Register_Control_LED_Persistence_Nbits  CountFracLen=0  CountSampTime=1
      settings: SourceProductBaseCode=HD
  Logical Operator : Logic  Operator=OR  AllPortsSameDT=off  OutDataTypeStr=boolean
  Relational Operator8 : RelationalOperator  Operator=<=  OutDataTypeStr=boolean  RndMeth=Nearest
  "LED_control " : Outport
  wires:
  Relational Operator8/1 -> Chart/2(count_reached)
  LED_trigger/1 -> Logical Operator/2, Chart/1(LED_trigger)
  Chart/1(LED_signal) -> "LED_control "/1
  "HDL Counter "/1 -> Relational Operator8/2
  LED_persistence_samples/1 -> Relational Operator8/1
  Chart/2(counter_reset) -> Logical Operator/1
  Logical Operator/1 -> "HDL Counter "/1

== system AD1939_Avalon_Stream_Processing_v1/DataPlane/Signal Energy LED Driver/Left Channel Processing/LED_Driver/Subsystem6 ==
  note: Don't start counter
      | as long as LED_trigger is asserted
  LED_trigger : Inport
  LED_persistence_samples : Inport  Port=2
  Chart : Stateflow chart  TreatAsAtomicUnit=on
  "HDL Counter " : hdlsllib/Sources/HDL Counter  CountType=Free running  CountInit=0  CountStep=1  CountMax=25  CountFromType=Initial value  CountFrom=0  CountResetPort=on  CountLoadPort=off  CountEnbPort=off  CountDirPort=off  CountDataType=Unsigned  CountWordLen=Register_Control_LED_Persistence_Nbits  CountFracLen=0  CountSampTime=1
      settings: SourceProductBaseCode=HD
  Logical Operator : Logic  Operator=OR  AllPortsSameDT=off  OutDataTypeStr=boolean
  Relational Operator8 : RelationalOperator  Operator=<=  OutDataTypeStr=boolean  RndMeth=Nearest
  "LED_control " : Outport
  wires:
  Relational Operator8/1 -> Chart/2(count_reached)
  LED_trigger/1 -> Logical Operator/2, Chart/1(LED_trigger)
  Chart/1(LED_signal) -> "LED_control "/1
  "HDL Counter "/1 -> Relational Operator8/2
  LED_persistence_samples/1 -> Relational Operator8/1
  Chart/2(counter_reset) -> Logical Operator/1
  Logical Operator/1 -> "HDL Counter "/1

== system AD1939_Avalon_Stream_Processing_v1/DataPlane/Signal Energy LED Driver/Left Channel Processing/LED_Driver/Subsystem7 ==
  note: Don't start counter
      | as long as LED_trigger is asserted
  LED_trigger : Inport
  LED_persistence_samples : Inport  Port=2
  Chart : Stateflow chart  TreatAsAtomicUnit=on
  "HDL Counter " : hdlsllib/Sources/HDL Counter  CountType=Free running  CountInit=0  CountStep=1  CountMax=25  CountFromType=Initial value  CountFrom=0  CountResetPort=on  CountLoadPort=off  CountEnbPort=off  CountDirPort=off  CountDataType=Unsigned  CountWordLen=Register_Control_LED_Persistence_Nbits  CountFracLen=0  CountSampTime=1
      settings: SourceProductBaseCode=HD
  Logical Operator : Logic  Operator=OR  AllPortsSameDT=off  OutDataTypeStr=boolean
  Relational Operator8 : RelationalOperator  Operator=<=  OutDataTypeStr=boolean  RndMeth=Nearest
  "LED_control " : Outport
  wires:
  Relational Operator8/1 -> Chart/2(count_reached)
  LED_trigger/1 -> Logical Operator/2, Chart/1(LED_trigger)
  Chart/1(LED_signal) -> "LED_control "/1
  "HDL Counter "/1 -> Relational Operator8/2
  LED_persistence_samples/1 -> Relational Operator8/1
  Chart/2(counter_reset) -> Logical Operator/1
  Logical Operator/1 -> "HDL Counter "/1

== stateflow chart AD1939_Avalon_Stream_Processing_v1/DataPlane/Signal Energy LED Driver/Left Channel Processing/LED_Driver/Subsystem/Chart ==
  settings: executeAtInitialization=1
  note: Turn on LED (LED_signal = true)
      | and start the counter when the LED_on state is entered.
      | When the counter reaches final count value, count_reach is asserted and
      | the state transitions to LED_off where the LED is turned off.
  state LED_on
    entry: LED_signal=true;
    entry: counter_reset=false;
  state LED_off
    entry: LED_signal=false;
    entry: counter_reset=true;
  note: Transition to state LED_on
      | when LED_trigger is asserted
  note: To update, parse chart to update signal names
      | Chart -> Parse Chart
      |
      | To add/remove/edit signals see:
      |  https://www.mathworks.com/help/stateflow/ug/using-the-model-explorer-with-stateflow-objects.html
  (default) -> LED_off
  LED_off -> LED_on : [LED_trigger == 1]
  LED_on -> LED_off [order 2] : [count_reached==1]
  LED_on -> LED_on [order 1] : [count_reached == 0]
  data: LED_trigger input; count_reached input; LED_signal output; counter_reset output

== stateflow chart AD1939_Avalon_Stream_Processing_v1/DataPlane/Signal Energy LED Driver/Left Channel Processing/LED_Driver/Subsystem1/Chart ==
  settings: executeAtInitialization=1
  note: Turn on LED (LED_signal = true)
      | and start the counter when the LED_on state is entered.
      | When the counter reaches final count value, count_reach is asserted and
      | the state transitions to LED_off where the LED is turned off.
  state LED_on
    entry: LED_signal=true;
    entry: counter_reset=false;
  state LED_off
    entry: LED_signal=false;
    entry: counter_reset=true;
  note: Transition to state LED_on
      | when LED_trigger is asserted
  note: To update, parse chart to update signal names
      | Chart -> Parse Chart
      |
      | To add/remove/edit signals see:
      |  https://www.mathworks.com/help/stateflow/ug/using-the-model-explorer-with-stateflow-objects.html
  (default) -> LED_off
  LED_off -> LED_on : [LED_trigger == 1]
  LED_on -> LED_off [order 2] : [count_reached==1]
  LED_on -> LED_on [order 1] : [count_reached == 0]
  data: LED_trigger input; count_reached input; LED_signal output; counter_reset output

== stateflow chart AD1939_Avalon_Stream_Processing_v1/DataPlane/Signal Energy LED Driver/Left Channel Processing/LED_Driver/Subsystem2/Chart ==
  settings: executeAtInitialization=1
  note: Turn on LED (LED_signal = true)
      | and start the counter when the LED_on state is entered.
      | When the counter reaches final count value, count_reach is asserted and
      | the state transitions to LED_off where the LED is turned off.
  state LED_on
    entry: LED_signal=true;
    entry: counter_reset=false;
  state LED_off
    entry: LED_signal=false;
    entry: counter_reset=true;
  note: Transition to state LED_on
      | when LED_trigger is asserted
  note: To update, parse chart to update signal names
      | Chart -> Parse Chart
      |
      | To add/remove/edit signals see:
      |  https://www.mathworks.com/help/stateflow/ug/using-the-model-explorer-with-stateflow-objects.html
  (default) -> LED_off
  LED_off -> LED_on : [LED_trigger == 1]
  LED_on -> LED_off [order 2] : [count_reached==1]
  LED_on -> LED_on [order 1] : [count_reached == 0]
  data: LED_trigger input; count_reached input; LED_signal output; counter_reset output

== stateflow chart AD1939_Avalon_Stream_Processing_v1/DataPlane/Signal Energy LED Driver/Left Channel Processing/LED_Driver/Subsystem3/Chart ==
  settings: executeAtInitialization=1
  note: Turn on LED (LED_signal = true)
      | and start the counter when the LED_on state is entered.
      | When the counter reaches final count value, count_reach is asserted and
      | the state transitions to LED_off where the LED is turned off.
  state LED_on
    entry: LED_signal=true;
    entry: counter_reset=false;
  state LED_off
    entry: LED_signal=false;
    entry: counter_reset=true;
  note: Transition to state LED_on
      | when LED_trigger is asserted
  note: To update, parse chart to update signal names
      | Chart -> Parse Chart
      |
      | To add/remove/edit signals see:
      |  https://www.mathworks.com/help/stateflow/ug/using-the-model-explorer-with-stateflow-objects.html
  (default) -> LED_off
  LED_off -> LED_on : [LED_trigger == 1]
  LED_on -> LED_off [order 2] : [count_reached==1]
  LED_on -> LED_on [order 1] : [count_reached == 0]
  data: LED_trigger input; count_reached input; LED_signal output; counter_reset output

== stateflow chart AD1939_Avalon_Stream_Processing_v1/DataPlane/Signal Energy LED Driver/Left Channel Processing/LED_Driver/Subsystem4/Chart ==
  settings: executeAtInitialization=1
  note: Turn on LED (LED_signal = true)
      | and start the counter when the LED_on state is entered.
      | When the counter reaches final count value, count_reach is asserted and
      | the state transitions to LED_off where the LED is turned off.
  state LED_on
    entry: LED_signal=true;
    entry: counter_reset=false;
  state LED_off
    entry: LED_signal=false;
    entry: counter_reset=true;
  note: Transition to state LED_on
      | when LED_trigger is asserted
  note: To update, parse chart to update signal names
      | Chart -> Parse Chart
      |
      | To add/remove/edit signals see:
      |  https://www.mathworks.com/help/stateflow/ug/using-the-model-explorer-with-stateflow-objects.html
  (default) -> LED_off
  LED_off -> LED_on : [LED_trigger == 1]
  LED_on -> LED_off [order 2] : [count_reached==1]
  LED_on -> LED_on [order 1] : [count_reached == 0]
  data: LED_trigger input; count_reached input; LED_signal output; counter_reset output

== stateflow chart AD1939_Avalon_Stream_Processing_v1/DataPlane/Signal Energy LED Driver/Left Channel Processing/LED_Driver/Subsystem5/Chart ==
  settings: executeAtInitialization=1
  note: Turn on LED (LED_signal = true)
      | and start the counter when the LED_on state is entered.
      | When the counter reaches final count value, count_reach is asserted and
      | the state transitions to LED_off where the LED is turned off.
  state LED_on
    entry: LED_signal=true;
    entry: counter_reset=false;
  state LED_off
    entry: LED_signal=false;
    entry: counter_reset=true;
  note: Transition to state LED_on
      | when LED_trigger is asserted
  note: To update, parse chart to update signal names
      | Chart -> Parse Chart
      |
      | To add/remove/edit signals see:
      |  https://www.mathworks.com/help/stateflow/ug/using-the-model-explorer-with-stateflow-objects.html
  (default) -> LED_off
  LED_off -> LED_on : [LED_trigger == 1]
  LED_on -> LED_off [order 2] : [count_reached==1]
  LED_on -> LED_on [order 1] : [count_reached == 0]
  data: LED_trigger input; count_reached input; LED_signal output; counter_reset output
